simulink model "M5_2301EE20_exp06_Uniplolar"  (R2024b)
settings: Solver=VariableStepAuto  StartTime=0.0  StopTime=1  RelTol=1e-3
libraries: spsIGBTLib x4, spsDCVoltageSourceLib x1, simulink x1, spsSeriesRLCBranchLib x1, spsVoltageMeasurementLib x1, sps_lib x1
settings Model: Creator=prasa  LastModifiedBy=prasa

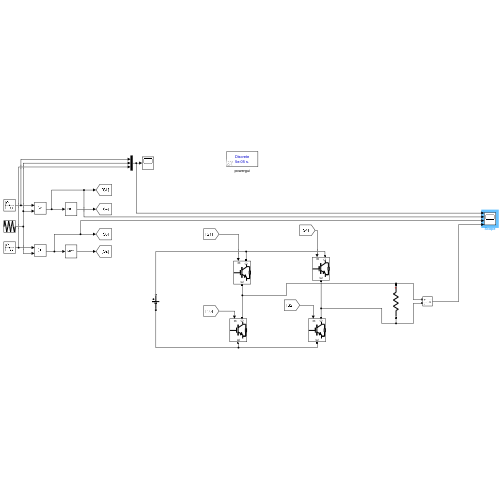
[thumbnail: Simulink's stored preview of the top-level diagram]
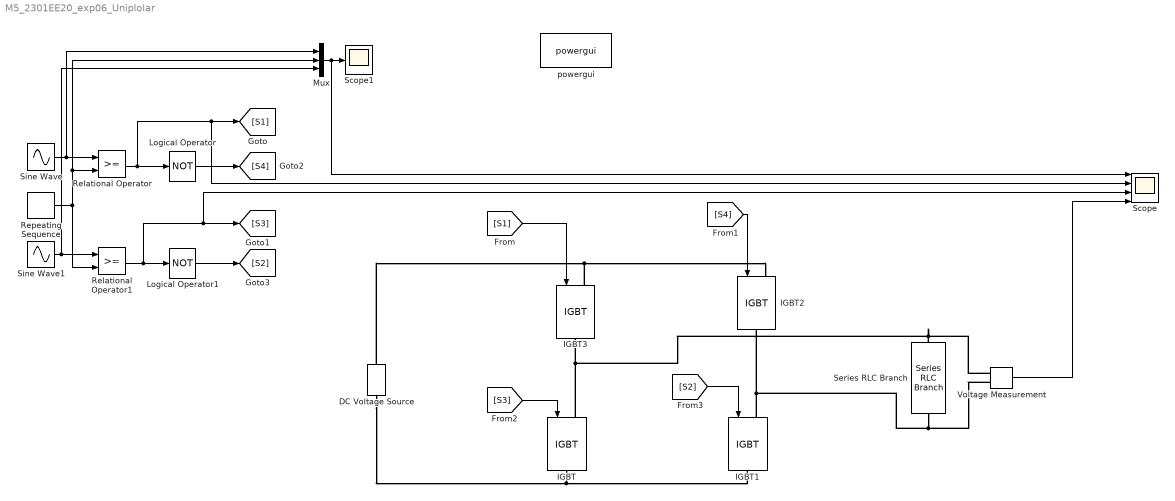
== system M5_2301EE20_exp06_Uniplolar ==
  DC Voltage Source : spsDCVoltageSourceLib/DC Voltage Source  Amplitude=100  Measurements=None
  IGBT{,1..3} (4 alike) : spsIGBTLib/IGBT  Ron=0.001  Lon=0  Vf=1  Tf=1e-6  Tt=2e-6  IC=0  Rs=1e5  Cs=inf  Measurements=off
  Logical Operator : Logic  Operator=NOT  AllPortsSameDT=off  OutDataTypeStr=boolean
  Logical Operator1 : Logic  Operator=NOT  AllPortsSameDT=off  OutDataTypeStr=boolean
  Mux : Mux  Inputs=3
  Relational Operator : RelationalOperator  OutDataTypeStr=boolean  RndMeth=Simplest  InputSameDT=off
  Relational Operator1 : RelationalOperator  OutDataTypeStr=boolean  RndMeth=Simplest  InputSameDT=off
  Repeating Sequence : simulink/Sources/Repeating Sequence  rep_seq_t=[0 1 2 3 4]*[1/400]  rep_seq_y=[0 1 0 -1 0]
  Scope : Scope  NumInputPorts=4
  Scope1 : Scope
  Series RLC Branch : spsSeriesRLCBranchLib/Series RLC Branch  LConnTagsString=__new0  RConnTagsString=__new0  BranchType=R  Resistance=10  Inductance=50e-3  SetiL0=off  InitialCurrent=0  Capacitance=1e-6  Setx0=off  InitialVoltage=0  Measurements=None
  Sine Wave : Sin  Frequency=2*pi*50  SampleTime=0
  Sine Wave1 : Sin  Frequency=2*pi*50  Phase=180  SampleTime=0
  Voltage Measurement : spsVoltageMeasurementLib/Voltage Measurement  PhasorSimulation=off  OutputType=Complex  PSBequivalent=0
  powergui : sps_lib/powergui  Priority=1  SimulationMode=Discrete  SampleTime=5e-5  frequency=60  Iterations=50  frequencyindice=0  Pbase=100e6  ErrMax=1e-4  UnitsV=kV  UnitsW=MW  buscounter=0  FunctionMessages=off  echomessages=off  EnableUseOfTLC=off  CurrentSourceSwitches=off  DisableSnubberDevices=off  DisableRonSwitches=off  DisableVfSwitches=off  DisplayEquations=off  AutomaticDiscreteSolvers=off  SolverType=Tustin/Backward Euler (TBE)  Interpol=off  ExternalGateDelay=off  methode=off  Ts=100  x0status=blocks  SPID=on  SwTol=0  HookPort=off  NonlinearTolerance=1e-4  nMaxIteration=100  ContinueOnMaxIteration=off  RestoreLinks=warning  ResistiveCurrentMeasurement=off  Frange=[0:2:500]  Ylog=off  Xlog=on  ShowGrid=off  save=off  variable=ZData  structure=0  ZoomFFT=off  StartTime=0.0  cycles=1  DisplayStyle=1  fundamental=60  FreqAxis=off  MaxFrequency=1000  frequencyindicesteady=1  RmsSteady=1  display=off
  wires:
  Repeating Sequence/1 -> Relational Operator1/2, Mux/2, Relational Operator/2
  Relational Operator/1 -> Scope/2, [S1], Logical Operator/1
  [S1] -> IGBT3/1
  Sine Wave/1 -> Mux/1, Relational Operator/1
  [S4] -> IGBT2/1
  [S2] -> IGBT1/1
  [S3] -> IGBT/1
  Sine Wave1/1 -> Mux/3, Relational Operator1/1
  Logical Operator/1 -> [S4]
  Logical Operator1/1 -> [S2]
  Relational Operator1/1 -> Scope/3, [S3], Logical Operator1/1
  Mux/1 -> Scope/1, Scope1/1
  Voltage Measurement/1 -> Scope/4
  connections:
  IGBT1/LConn1 -- Voltage Measurement/LConn2 -- Series RLC Branch/RConn1 -- IGBT2/RConn1
  IGBT/LConn1 -- Series RLC Branch/LConn1 -- Voltage Measurement/LConn1 -- IGBT3/RConn1
  IGBT3/LConn1 -- DC Voltage Source/RConn1 -- IGBT2/LConn1
  IGBT/RConn1 -- DC Voltage Source/LConn1 -- IGBT1/RConn1
